simulink model "single_phase_PVarry_inverter"  (Simulink 8.3)
settings: Solver=ode23tb  StartTime=0.0  StopTime=0.1  RelTol=1e-3
undefined symbols (not defined in the file or in its folder): Newton, Raphson
libraries: powerlib x15, powerlib_extras x1, simulink x1
settings Model: Creator=????  LastModifiedBy=jt  SimulationMode=accelerator
settings OptimizationCC: ExpressionDepthLimit=2147483647  InitFltsAndDblsToZero=on
settings DebuggingCC: MaxConsecutiveZCsMsg=none  FcnCallInpInsideContextMsg=UseLocalSettings

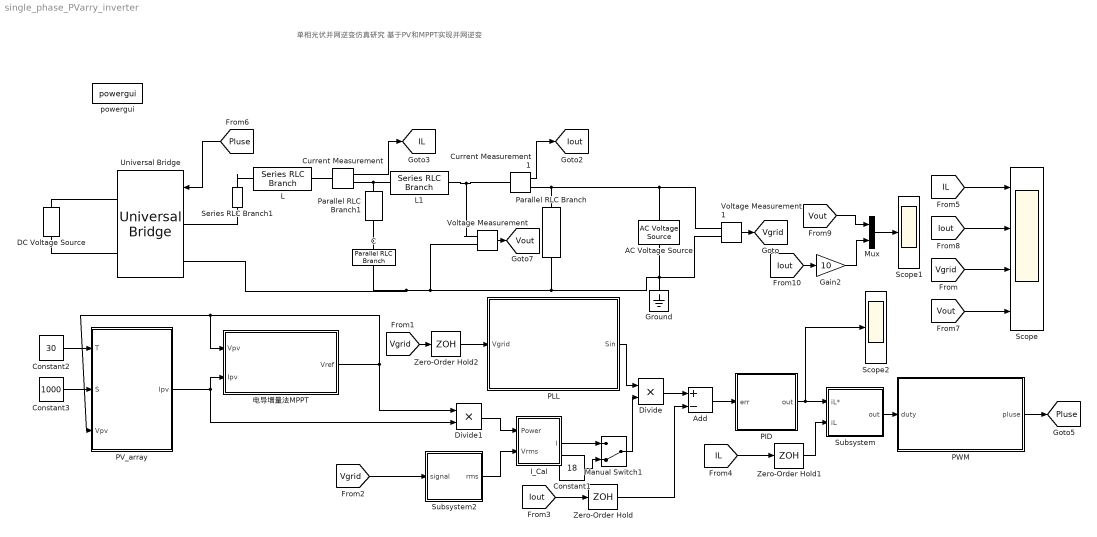
== system single_phase_PVarry_inverter ==
  note: 单相光伏并网逆变仿真研究
      | 基于PV和MPPT实现并网逆变
  AC Voltage Source : powerlib/Electrical Sources/AC Voltage Source  Amplitude=311  Phase=0  Frequency=50  SampleTime=0  Measurements=None
  Add : Sum  Inputs=+-
  C : powerlib/Elements/Parallel RLC Branch  LConnTagsString=a  RConnTagsString=__new0  BranchType=C  Resistance=6  Inductance=7e-3  SetiL0=off  InitialCurrent=0  Capacitance=6e-6  Setx0=off  InitialVoltage=0  Measurements=None
  Constant1 : Constant  Value=18
  Constant2 : Constant  Value=30
  Constant3 : Constant  Value=1000
  Current Measurement : powerlib/Measurements/Current Measurement  PhasorSimulation=off  OutputType=Complex  PSBequivalent=0
  Current Measurement1 : powerlib/Measurements/Current Measurement  PhasorSimulation=off  OutputType=Complex  PSBequivalent=0
  DC Voltage Source : powerlib/Electrical Sources/DC Voltage Source  Amplitude=400  Measurements=None
  Divide : Product  Inputs=**
  Divide1 : Product
  Gain2 : Gain  Gain=10
  Ground : powerlib/Elements/Ground  LConnTagsString=a
  I_Cal : Subsystem
  L : powerlib/Elements/Series RLC Branch  LConnTagsString=__new0  RConnTagsString=__new0  BranchType=L  Resistance=1  Inductance=6e-3  SetiL0=off  InitialCurrent=0  Capacitance=1e-6  Setx0=off  InitialVoltage=0  Measurements=None
  L1 : powerlib/Elements/Series RLC Branch  LConnTagsString=__new0  RConnTagsString=__new0  BranchType=L  Resistance=1  Inductance=1e-6  SetiL0=off  InitialCurrent=0  Capacitance=1e-6  Setx0=off  InitialVoltage=0  Measurements=None
  Manual Switch1 : ManualSwitch  CurrentSetting=0
  Mux : Mux  Inputs=2
  PID : Subsystem  mask{P=0.1, I=800, D=0}
      mask prompts: P "Proportional"; I "Integral"; D "Derivative"
      mask Display: disp('PID')
  PLL : Subsystem
      mask Display: disp('PLL')
  PV_array : Subsystem  mask{a=0.015, b=0.7, Sref=1000, Rs=2, Isc=5, Voc=300, Vm=220, Im=4.5, Tref=25}
      mask Display: disp('PV_array')
  PWM : Subsystem
      mask Display: disp('PWM')
  Parallel RLC Branch : powerlib/Elements/Parallel RLC Branch  LConnTagsString=a  RConnTagsString=__new0  BranchType=R  Resistance=100  Inductance=1e-3  SetiL0=off  InitialCurrent=0  Capacitance=1e-6  Setx0=off  InitialVoltage=0  Measurements=None
  Parallel RLC Branch1 : powerlib/Elements/Parallel RLC Branch  LConnTagsString=a  RConnTagsString=__new0  BranchType=R  Resistance=0.05  Inductance=1e-3  SetiL0=off  InitialCurrent=0  Capacitance=1e-6  Setx0=off  InitialVoltage=0  Measurements=None
  Scope : Scope  NumInputPorts=4
      settings: YMin=-20~-20~-350~-350  YMax=20~20~350~350  SampleInput=on
  Scope1 : Scope
      settings: YMin=-6000  YMax=5500  SampleInput=on
  Scope2 : Scope
      settings: YMin=-2.25  YMax=0.5  SaveName=ScopeData2  SampleInput=on
  Series RLC Branch1 : powerlib/Elements/Series RLC Branch  LConnTagsString=__new0  RConnTagsString=__new0  BranchType=R  Resistance=0.01  Inductance=1e-3  SetiL0=off  InitialCurrent=0  Capacitance=1e-6  Setx0=off  InitialVoltage=0  Measurements=None
  Subsystem : Subsystem
  Subsystem2 : Subsystem  mask{f=50}
      mask prompts: f "Fundamental frequency (Hz)"
      mask Display: disp('RMS')
  Universal Bridge : powerlib/Power Electronics/Universal Bridge  Arms=2  SnubberResistance=1e5  SnubberCapacitance=inf  Device=IGBT / Diodes  Ron=1e-3  Lon=0  ForwardVoltages="[  0  0  ]"  ForwardVoltage=0  GTOparameters=[ 10e-6 , 20e-6 ]  IGBTparameters=[ 1e-6 , 2e-6 ]  Measurements=None  Measurements_2=None  converterType=Rectifier
  Voltage Measurement : powerlib/Measurements/Voltage Measurement  PhasorSimulation=off  OutputType=Complex  PSBequivalent=0
  Voltage Measurement1 : powerlib/Measurements/Voltage Measurement  PhasorSimulation=off  OutputType=Complex  PSBequivalent=0
  Zero-Order Hold : ZeroOrderHold  SampleTime=1e-5
  Zero-Order Hold1 : ZeroOrderHold  SampleTime=1e-5
  Zero-Order Hold2 : ZeroOrderHold  SampleTime=1e-5
  powergui : powerlib/powergui  SimulationMode=Continuous  SolverType=Tustin  SampleTime=1e-10  frequency=60  SPID=off  DisableSnubberDevices=off  DisableRonSwitches=off  DisableVfSwitches=off  SwTol=0  Interpol=off  DisplayEquations=off  Ts=0  methode=off  frequencyindice=50  Pbase=100e6  ErrMax=1e-4  Iterations=50  UnitsV=kV  UnitsW=MW  FunctionMessages=off  echomessages=off  HookPort=off  EnableUseOfTLC=off  x0status=blocks  RestoreLinks=warning  ResistiveCurrentMeasurement=off  Frange=[0:2:500]  Ylog=off  Xlog=on  ShowGrid=off  save=off  variable=ZData  structure=ScopeData  ZoomFFT=off  StartTime=0.0  cycles=1  DisplayStyle=1  fundamental=60  FreqAxis=off  MaxFrequency=1000  frequencyindicesteady=1  RmsSteady=1  display=off
  电导增量法MPPT : Subsystem
      mask Display: disp('PV_array_MPPT')
  tag scope: IL=global, Iout=global, Pluse=global, Vgrid=global, Vout=global
  wires:
  Current Measurement1/1 -> [Iout]
  Constant3/1 -> PV_array/2(S)
  Constant2/1 -> PV_array/1(T)
  [Vgrid] -> Scope/3
  Voltage Measurement1/1 -> [Vgrid]
  [Iout] -> Zero-Order Hold/1
  Current Measurement/1 -> [IL]
  [IL] -> Scope/1
  [Pluse] -> Universal Bridge/1
  Voltage Measurement/1 -> [Vout]
  [Vout] -> Scope/4
  [Iout] -> Scope/2
  Divide1/1 -> I_Cal/1(Power)
  Subsystem2/1(rms) -> I_Cal/2(Vrms)
  PLL/1(Sin) -> Divide/1
  Divide/1 -> Add/1
  Zero-Order Hold/1 -> Add/2
  Add/1 -> PID/1(err)
  PID/1(out) -> Scope2/1, Subsystem/1(iL*)
  Subsystem/1(out) -> PWM/1(duty)
  PWM/1(pluse) -> [Pluse]
  Mux/1 -> Scope1/1
  [Vout] -> Mux/1
  [Iout] -> Gain2/1
  Gain2/1 -> Mux/2
  电导增量法MPPT/1(Vref) -> Divide1/1, 电导增量法MPPT/1(Vpv), PV_array/3(Vpv)
  PV_array/1(Ipv) -> 电导增量法MPPT/2(Ipv), Divide1/2
  Zero-Order Hold2/1 -> PLL/1(Vgrid)
  [IL] -> Zero-Order Hold1/1
  Zero-Order Hold1/1 -> Subsystem/2(iL)
  [Vgrid] -> Zero-Order Hold2/1
  [Vgrid] -> Subsystem2/1(signal)
  I_Cal/1(I) -> Manual Switch1/1
  Manual Switch1/1 -> Divide/2
  Constant1/1 -> Manual Switch1/2
  connections:
  L/RConn1 -- Current Measurement/LConn1
  Current Measurement1/RConn1 -- Parallel RLC Branch/LConn1 -- AC Voltage Source/RConn1 -- Voltage Measurement1/LConn1
  Universal Bridge/LConn2 -- C/RConn1 -- Voltage Measurement/LConn2 -- Parallel RLC Branch/RConn1 -- Voltage Measurement1/LConn2 -- AC Voltage Source/LConn1 -- Ground/LConn1
  Voltage Measurement/LConn1 -- Current Measurement1/LConn1 -- L1/RConn1
  Universal Bridge/LConn1 -- Series RLC Branch1/LConn1
  Series RLC Branch1/RConn1 -- L/LConn1
  Universal Bridge/RConn1 -- DC Voltage Source/RConn1
  Universal Bridge/RConn2 -- DC Voltage Source/LConn1
  Parallel RLC Branch1/LConn1 -- C/LConn1
  Current Measurement/RConn1 -- L1/LConn1 -- Parallel RLC Branch1/RConn1

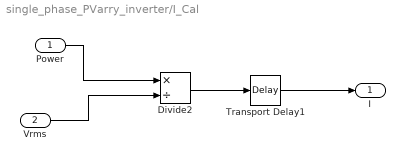
== system single_phase_PVarry_inverter/I_Cal ==
  Power : Inport
  Vrms : Inport  Port=2
  Divide2 : Product  Inputs=*/
  Transport Delay1 : TransportDelay  DelayTime=1e-5  BufferSize=2048
  I : Outport
  wires:
  Power/1 -> Divide2/1
  Vrms/1 -> Divide2/2
  Divide2/1 -> Transport Delay1/1
  Transport Delay1/1 -> I/1

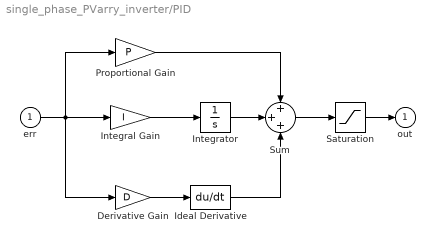
== system single_phase_PVarry_inverter/PID ==
  err : Inport
  Derivative Gain : Gain  Gain=D  SaturateOnIntegerOverflow=on  OutDataTypeStr=Inherit: Same as input  ParamDataTypeStr=Inherit: Same as input
  Ideal Derivative : Derivative
  Integral Gain : Gain  Gain=I  SaturateOnIntegerOverflow=on  OutDataTypeStr=Inherit: Same as input  ParamDataTypeStr=Inherit: Same as input
  Integrator : Integrator
  Proportional Gain : Gain  Gain=P  SaturateOnIntegerOverflow=on  OutDataTypeStr=Inherit: Same as input  ParamDataTypeStr=Inherit: Same as input
  Saturation : Saturate  UpperLimit=50  LowerLimit=-50
  Sum : Sum  Inputs=+++  SaturateOnIntegerOverflow=on  InputSameDT=on  OutDataTypeStr=Inherit: Same as first input
  out : Outport  InitialOutput=0
  wires:
  Proportional Gain/1 -> Sum/1
  Integral Gain/1 -> Integrator/1
  err/1 -> Proportional Gain/1, Integral Gain/1, Derivative Gain/1
  Integrator/1 -> Sum/2
  Ideal Derivative/1 -> Sum/3
  Derivative Gain/1 -> Ideal Derivative/1
  Sum/1 -> Saturation/1
  Saturation/1 -> out/1

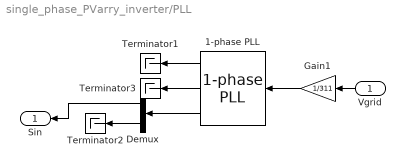
== system single_phase_PVarry_inverter/PLL ==
  Vgrid : Inport
  1-phase PLL : powerlib_extras/Control  Blocks/1-phase PLL  Par_Init=[0 50]  ParK=[50 80 0]  AGC=off
  Demux : Demux  Outputs=2
  Gain1 : Gain  Gain=1/311
  Terminator1 : Terminator
  Terminator2 : Terminator
  Terminator3 : Terminator
  Sin : Outport
  wires:
  Demux/2 -> Terminator2/1
  1-phase PLL/3 -> Demux/1
  Demux/1 -> Sin/1
  1-phase PLL/2 -> Terminator3/1
  1-phase PLL/1 -> Terminator1/1
  Vgrid/1 -> Gain1/1
  Gain1/1 -> 1-phase PLL/1

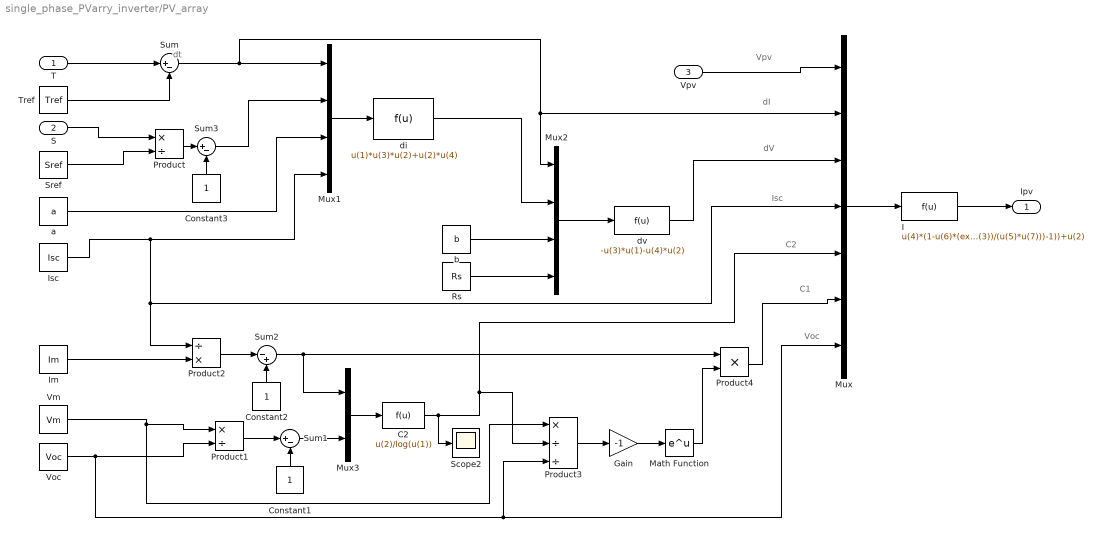
== system single_phase_PVarry_inverter/PV_array ==
  note: Vpv
  note: Voc
  note: C1
  note: C2
  note: Isc
  note: dV
  note: dI
  note: dt
  T : Inport
  S : Inport  Port=2
  Vpv : Inport  Port=3
  C2 : Fcn  Expr=u(2)/log(u(1))
  Constant1 : Constant
  Constant2 : Constant
  Constant3 : Constant
  Gain : Gain  Gain=-1
  I : Fcn  Expr=u(4)*(1-u(6)*(exp((u(1)-u(3))/(u(5)*u(7)))-1))+u(2)
  Im : Constant  Value=Im
  Isc : Constant  Value=Isc
  Math Function : Math  SaturateOnIntegerOverflow=on
  Mux : Mux  Inputs=7
  Mux1 : Mux
  Mux2 : Mux
  Mux3 : Mux  Inputs=2
  Product : Product  Inputs=*/  RndMeth=Zero
  Product1 : Product  Inputs=*/  RndMeth=Zero
  Product2 : Product  Inputs=/*  RndMeth=Zero
  Product3 : Product  Inputs=*//  RndMeth=Zero
  Product4 : Product  Inputs=**  RndMeth=Zero
  Rs : Constant  Value=Rs
  Scope2 : Scope
      settings: SaveName=ScopeData4
  Sref : Constant  Value=Sref
  Sum : Sum  Inputs=|+-
  Sum1 : Sum  Inputs=|+-
  Sum2 : Sum  Inputs=|-+
  Sum3 : Sum  Inputs=|+-
  Tref : Constant  Value=Tref
  Vm : Constant  Value=Vm
  Voc : Constant  Value=Voc
  a : Constant  Value=a
  b : Constant  Value=b
  di : Fcn  Expr=u(1)*u(3)*u(2)+u(2)*u(4)
  dv : Fcn  Expr=-u(3)*u(1)-u(4)*u(2)
  Ipv : Outport
  wires:
  Product4/1 -> Mux/6
  Math Function/1 -> Product4/2
  Gain/1 -> Math Function/1
  Product3/1 -> Gain/1
  Sum3/1 -> Mux1/2
  Constant3/1 -> Sum3/2
  Product/1 -> Sum3/1
  S/1 -> Product/1
  I/1 -> Ipv/1
  dv/1 -> Mux/3
  Vpv/1 -> Mux/1
  Mux/1 -> I/1
  C2/1 -> Product3/2, Mux/5, Scope2/1
  Sum1/1 -> Mux3/2
  Sum2/1 -> Mux3/1, Product4/1
  Im/1 -> Product2/2
  Constant1/1 -> Sum1/2
  Product1/1 -> Sum1/1
  Voc/1 -> Product1/2, Product3/3, Mux/7
  Vm/1 -> Product1/1, Product3/1
  Constant2/1 -> Sum2/2
  Product2/1 -> Sum2/1
  Mux3/1 -> C2/1
  Mux2/1 -> dv/1
  di/1 -> Mux2/2
  b/1 -> Mux2/3
  Mux1/1 -> di/1
  Isc/1 -> Mux1/4, Product2/1, Mux/4
  a/1 -> Mux1/3
  Sum/1 -> Mux1/1, Mux2/1, Mux/2
  Sref/1 -> Product/2
  Tref/1 -> Sum/2
  T/1 -> Sum/1
  Rs/1 -> Mux2/4

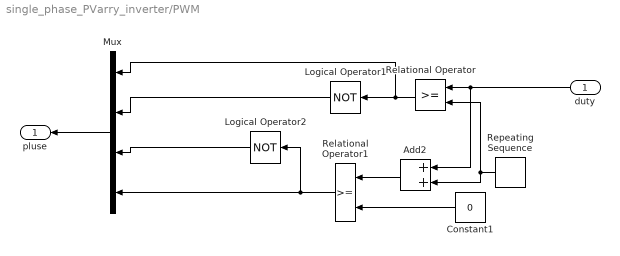
== system single_phase_PVarry_inverter/PWM ==
  duty : Inport
  Add2 : Sum
  Constant1 : Constant  Value=0
  Logical Operator1 : Logic  Operator=NOT  Inputs=1  AllPortsSameDT=off  OutDataTypeStr=boolean
  Logical Operator2 : Logic  Operator=NOT  Inputs=1  AllPortsSameDT=off  OutDataTypeStr=boolean
  Mux : Mux
  Relational Operator : RelationalOperator  OutDataTypeStr=boolean
  Relational Operator1 : RelationalOperator  OutDataTypeStr=boolean
  Repeating Sequence : simulink/Sources/Repeating Sequence  rep_seq_t=[0 1/40e3 1/20e3]  rep_seq_y=[-10 0 10]
  pluse : Outport
  wires:
  Add2/1 -> Relational Operator1/1
  Relational Operator/1 -> Logical Operator1/1, Mux/1
  Constant1/1 -> Relational Operator1/2
  Repeating Sequence/1 -> Relational Operator/2, Add2/2
  Logical Operator1/1 -> Mux/2
  duty/1 -> Relational Operator/1, Add2/1
  Relational Operator1/1 -> Mux/4, Logical Operator2/1
  Mux/1 -> pluse/1
  Logical Operator2/1 -> Mux/3

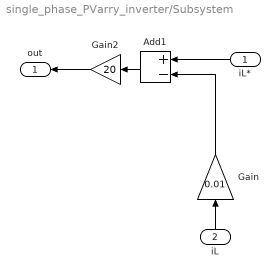
== system single_phase_PVarry_inverter/Subsystem ==
  iL* : Inport
  iL : Inport  Port=2
  Add1 : Sum  Inputs=+-
  Gain : Gain  Gain=0.01
  Gain2 : Gain  Gain=20
  out : Outport
  wires:
  Add1/1 -> Gain2/1
  iL*/1 -> Add1/1
  Gain/1 -> Add1/2
  Gain2/1 -> out/1
  iL/1 -> Gain/1

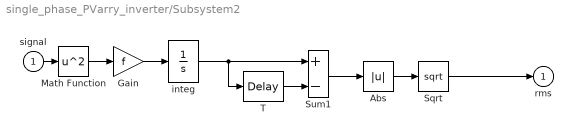
== system single_phase_PVarry_inverter/Subsystem2 ==
  signal : Inport
  Abs : Abs  SaturateOnIntegerOverflow=on
  Gain : Gain  Gain=f  SaturateOnIntegerOverflow=on  OutDataTypeStr=Inherit: Same as input  ParamDataTypeStr=Inherit: Same as input
  Math Function : Math  Operator=square  SaturateOnIntegerOverflow=on
  Sqrt : Sqrt  AlgorithmType=Newton-Raphson  SaturateOnIntegerOverflow=on
  Sum1 : Sum  Inputs=+-  SaturateOnIntegerOverflow=on  InputSameDT=on  OutDataTypeStr=Inherit: Same as first input
  T : TransportDelay  DelayTime=1/f  BufferSize=2048
  integ : Integrator
  rms : Outport  InitialOutput=0
  wires:
  Sum1/1 -> Abs/1
  signal/1 -> Math Function/1
  Math Function/1 -> Gain/1
  Gain/1 -> integ/1
  T/1 -> Sum1/2
  Abs/1 -> Sqrt/1
  Sqrt/1 -> rms/1
  integ/1 -> T/1, Sum1/1

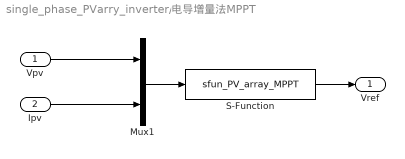
== system single_phase_PVarry_inverter/电导增量法MPPT ==
  Vpv : Inport
  Ipv : Inport  Port=2
  Mux1 : Mux  Inputs=2
  S-Function : S-Function  FunctionName=sfun_PV_array_MPPT  EnableBusSupport=off
  Vref : Outport
  wires:
  S-Function/1 -> Vref/1
  Ipv/1 -> Mux1/2
  Mux1/1 -> S-Function/1
  Vpv/1 -> Mux1/1
